simulink model "sim_final_VSS_PWM"  (R2019a)
settings: Solver=FixedStepAuto  StartTime=0.0  StopTime=end_time  FixedStep=1e-3  RelTol=1e-3  EnableMultiTasking=on
values from neighbouring files (symbols this model uses):
  a = 47    [mod1s.m]
  b = -35    [mod1s.m]
  C1 = 0.76    [mod1s.m]
  C2 = 11    [mod1s.m]
  d = 0.5    [mod1s.m]
  ds = 1    [mod1s.m]
  h = 4    [mod1s.m]
  K = 19    [mod1s.m]
  k1 = 3    [mod1s.m]
  k2 = 40    [mod1s.m]
  T = 29    [mod1s.m]
  x0 = -100    [mod1s.m]
  y0 = 0    [mod1s.m]
  z0 = 0    [mod1s.m]
undefined symbols (not defined in the file or in its folder): zad
libraries: simulink x2, simulink_extras x1
settings Model: Creator=user  LastModifiedBy=ogure
settings SolverCC: SolverResetMethod=Robust
settings DataIOCC: LimitDataPoints=on  MaxDataPoints=1000000  SaveFormat=Array  ReturnWorkspaceOutputs=off  OutputSaveName=X
settings OptimizationCC: LifeSpan=inf
settings DebuggingCC: SolverPrmCheckMsg=warning  SFUnexpectedBacktrackingDiag=warning  SFNoUnconditionalDefaultTransitionDiag=warning  SFExecutionAtInitializationDiag=none  ArithmeticOperatorsInVariantConditions=warning
settings HardwareCC: ProdBitPerPointer=32  ProdBitPerSizeT=32  ProdBitPerPtrDiffT=32  ProdLargestAtomicFloat=None  ProdIntDivRoundTo=Undefined  ProdEndianess=Unspecified  ProdWordSize=32  ProdHWDeviceType=32-bit Generic
settings ModelReferenceCC: PropagateSignalLabelsOutOfModel=off
settings SFSimCC: SimUseLocalCustomCode=off
settings RTWCC: RTWUseLocalCustomCode=off
settings CodeAppCC: StateflowObjectComments=on
settings GRTTargetCC: TargetLangStandard=C89/C90 (ANSI)  GeneratePreprocessorConditionals=Disable all
settings ConfigComp: CovMetricSettings=dw  CovHtmlReporting=on  CovSaveCumulativeToWorkspaceVar=on  CovSaveSingleToWorkspaceVar=on  CovExternalEMLEnable=off  CovSFcnEnable=off

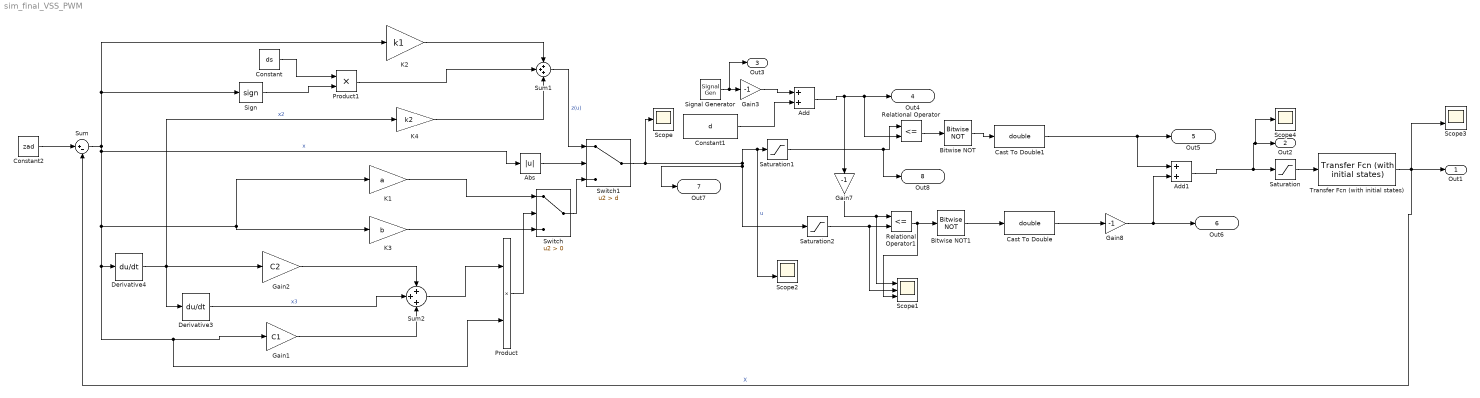
== system sim_final_VSS_PWM ==
  Abs : Abs
  Add : Sum
  Add1 : Sum
  Bitwise NOT : simulink/Logic and Bit Operations/Bitwise Operator  logicop=NOT  UseBitMask=off  BitMask=bin2dec('11011001')  BitMaskRealWorld=Stored Integer
  Bitwise NOT1 : simulink/Logic and Bit Operations/Bitwise Operator  logicop=NOT  UseBitMask=off  BitMask=bin2dec('11011001')  BitMaskRealWorld=Stored Integer
  Cast To Double : DataTypeConversion  OutDataTypeStr=double
  Cast To Double1 : DataTypeConversion  OutDataTypeStr=double
  Constant : Constant  Value=ds
  Constant1 : Constant  Value=d
  Constant2 : Constant  Value=zad
  Derivative3 : Derivative  CoefficientInTFapproximation=0.00000001
  Derivative4 : Derivative  CoefficientInTFapproximation=0.00000001
  Gain1 : Gain  Gain=C1
  Gain2 : Gain  Gain=C2
  Gain3 : Gain  Gain=-1
  Gain7 : Gain  Gain=-1
  Gain8 : Gain  Gain=-1
  K1 : Gain  Gain=a
  K2 : Gain  Gain=k1
  K3 : Gain  Gain=b
  K4 : Gain  Gain=k2
  Product : Product
  Product1 : Product
  Relational Operator : RelationalOperator  Operator=<=  OutDataTypeStr=boolean  ZeroCross=off  RndMeth=Simplest
  Relational Operator1 : RelationalOperator  Operator=<=  OutDataTypeStr=boolean  ZeroCross=off  RndMeth=Simplest
  Saturation : Saturate  UpperLimit=d  LowerLimit=-d
  Saturation1 : Saturate  UpperLimit=d  LowerLimit=-d
  Saturation2 : Saturate  UpperLimit=d  LowerLimit=-d
  Scope : Scope
  Scope1 : Scope  NumInputPorts=3
  Scope2 : Scope  NumInputPorts=2
  Scope3 : Scope  NumInputPorts=2
  Scope4 : Scope
  Sign : Signum
  Signal Generator : SignalGenerator  WaveForm=sawtooth  Amplitude=d  Frequency=10
  Sum : Sum  Inputs=|+-
  Sum1 : Sum  Inputs=+++
  Sum2 : Sum  Inputs=+++
  Switch : Switch  Criteria=u2 > Threshold  ZeroCross=off
  Switch1 : Switch  Criteria=u2 > Threshold  Threshold=d  ZeroCross=off
  Transfer Fcn (with initial states) : simulink_extras/Additional Linear/Transfer Fcn (with initial states)  N=K  D=[T^2 2*h*T 1 0]  X0=[z0 y0 x0]
  Out1 : Outport  SignalName=X
  Out2 : Outport  Port=2  SignalName=PWm
  Out3 : Outport  Port=3  SignalName=saw
  Out4 : Outport  Port=4  SignalName=sawnew
  Out5 : Outport  Port=5  SignalName=pwm1
  Out6 : Outport  Port=6  SignalName=pwm2
  Out7 : Outport  Port=7  SignalName=upr
  Out8 : Outport  Port=8  SignalName=upr_ogr
  wires:
  Transfer Fcn (with initial states)/1 -> Scope3/2, Sum/2, Out1/1  "X"
  Derivative3/1 -> Sum2/2  "x3"
  Gain1/1 -> Sum2/3
  Sum2/1 -> Product/1
  K1/1 -> Switch/1
  Sum/1 -> Abs/1, K1/1, K3/1, Gain1/1, Product/2, Derivative4/1, K2/1, Sign/1  "x"
  Derivative4/1 -> K4/1, Gain2/1, Derivative3/1  "x2"
  Product/1 -> Switch/2
  Gain2/1 -> Sum2/1
  K3/1 -> Switch/3
  Switch/1 -> Switch1/3
  Sign/1 -> Product1/2
  Constant/1 -> Product1/1
  K2/1 -> Sum1/1
  K4/1 -> Sum1/3
  Product1/1 -> Sum1/2
  Constant2/1 -> Sum/1
  Sum1/1 -> Switch1/1  "z(u)"
  Abs/1 -> Switch1/2
  Cast To Double1/1 -> Add1/1, Out5/1
  Gain8/1 -> Out6/1, Add1/2
  Relational Operator/1 -> Bitwise NOT/1
  Add1/1 -> Scope4/1, Out2/1, Saturation/1
  Cast To Double/1 -> Gain8/1
  Saturation1/1 -> Out8/1, Relational Operator/1
  Saturation2/1 -> Scope1/2, Relational Operator1/2
  Gain7/1 -> Scope1/1, Relational Operator1/1
  Relational Operator1/1 -> Scope1/3, Bitwise NOT1/1
  Gain3/1 -> Add/1
  Bitwise NOT/1 -> Cast To Double1/1
  Add/1 -> Out4/1, Relational Operator/2, Gain7/1
  Constant1/1 -> Add/2
  Signal Generator/1 -> Out3/1, Gain3/1
  Bitwise NOT1/1 -> Cast To Double/1
  Switch1/1 -> Scope/1, Out7/1, Saturation2/1, Scope2/2, Saturation1/1  "u"
  Saturation/1 -> Transfer Fcn (with initial states)/1
